simulink model "Ford_T3T6_ArchCnctnDigrm"  (R2016b)
settings: Solver=FixedStepDiscrete  StartTime=0.0  StopTime=10.0  RelTol=1e-3  EnableMultiTasking=on
libraries: canmsglib x15
(part 11 of 15)

== system Ford_T3T6_ArchCnctnDigrm/Vehicle Com/Rx Messages/Ambient Temperature ==
  note: FordVehOutdAirTVld Signal Required
  note: From COM
  MM078A_FordMsg41ABusHiSpd : Subsystem  Tag=4.0.X  Description=The purpose of the Ford Message 41A Bus High Speed function is to provide the Electric Power Steering system with vehicle odometer, climate, and Trailer Back Up Assist signals from CAN. The Ford Message 41A function will perform the missing message and signal invalid diagnostics as well as provide a validity signal for the signal values and received message.
      settings: AttributesFormatString=Version: %<Tag>
  Outside_Air_Temp_Stat : Ground
  tag scope: ComIPduCallout_Climate_Control_Data_FD1=global, ComTimeoutNotification_Outside_Air_Temp_Stat=global, FordVehOutdAirT=global, FordVehOutdAirTRaw=global
  wires:
  [ClrDiagcFlgProxy] -> MM078A_FordMsg41ABusHiSpd/1(ClrDiagcFlgProxy)
  [FordCanDtcInhb] -> MM078A_FordMsg41ABusHiSpd/2(FordCanDtcInhb)
  [FordEpsLifeCycMod] -> MM078A_FordMsg41ABusHiSpd/3(FordEpsLifeCycMod)
  Outside_Air_Temp_Stat/1 -> MM078A_FordMsg41ABusHiSpd/4(Ford_Outside_Air_Temp_Stat)
  [GetRefTmr100MicroSec32bit] -> MM078A_FordMsg41ABusHiSpd/5(GetRefTmr100MicroSec32bit)
  [GetTiSpan100MicroSec32bit] -> MM078A_FordMsg41ABusHiSpd/6(GetTiSpan100MicroSec32bit)
  [SetNtcSts] -> MM078A_FordMsg41ABusHiSpd/7(SetNtcSts)
  MM078A_FordMsg41ABusHiSpd/1(FordVehOutdAirT) -> [FordVehOutdAirT]
  MM078A_FordMsg41ABusHiSpd/2(FordVehOutdAirTRaw) -> [FordVehOutdAirTRaw]
  MM078A_FordMsg41ABusHiSpd/3(ComIPduCallout_Climate_Control_Data_FD1) -> [ComIPduCallout_Climate_Control_Data_FD1]
  MM078A_FordMsg41ABusHiSpd/4(ComTimeoutNotification_Outside_Air_Temp_Stat) -> [ComTimeoutNotification_Outside_Air_Temp_Stat]

== system Ford_T3T6_ArchCnctnDigrm/Vehicle Com/Rx Messages/Brake Data ==
  note: From COM
  note: From COM
  note: From COM
  note: From COM
  BrkTot_Tq_Actl : Ground
  Ground : Ground
  Ground6 : Ground
  Ground7 : Ground
  MM052A_FordMsg07DBusHiSpd : Subsystem  Tag=4.0.X  Description=The purpose of the Ford Message 07D Bus High Speed function is to provide the Electric Power Steering system with signal values for the Brake Oscillation Reduction and Trailer Back Up Assist function from CAN. The Ford Message 07D function will perform the missing message diagnostic, signal invalid diagnostic, and provide a validity flag for the received message and signal values.
      settings: AttributesFormatString=Version: %<Tag>
  MM058A_FordMsg165BusHiSpd : Subsystem  Tag=4.0.X  Description=The purpose of the Ford Message 165 Bus High Speed function is to provide the Electric Power Steering system with signal values for the EAC feature. The Ford Message 165 function will perform the missing message and signal invalid diagnostics.
      settings: AttributesFormatString=Version: %<Tag>
  MM063A_FordMsg213BusHiSpd : Subsystem  Tag=4.0.X  Description=The purpose of the Ford Message 213 Bus High Speed function is toprovide the Electric Power Steering system with signal values forthe Brake Oscillation Reduction, Lane Detection Warning, LKA, Traffic Jam Assist and Lane Center Assist functions from CAN.The FordMessage 213 function will perform the missing message and signal ivalid diagnostics as well as provide a validity flag for the signal values and received message.
      settings: AttributesFormatString=Version: %<Tag>
  MM077A_FordMsg415BusHiSpd : Subsystem  Tag=4.0.X  Description=The purpose of the Ford Message 415 Bus High Speed function is to provide the Electric Power Steering systemwith signal values for vehicle speed and the Trailer Back Up Assist function from CAN. The Ford Message 415function will perform the missing message and signal invalid diagnostics as well as provide a validity signalfor the signal values and received message.
      settings: AttributesFormatString=Version: %<Tag>
  VehVertComp_A_Actl : Ground
  tag scope: ComIPduCallout_BrakeSnData_4_FD1=global, ComIPduCallout_BrakeSysFeatures_FD1=global, ComIPduCallout_DesiredTorqBrk_FD1=global, ComIPduCallout_EngBrakeData_FD1=global, ComTimeoutNotification_BpedDrvAppl_D_Actl=global, ComTimeoutNotification_BrkTot_Tq_Actl=global, ComTimeoutNotification_CmbbDeny_B_ActlBrk=global, ComTimeoutNotification_Veh_V_ActlBrk=global, FordVehAbsActv=global, FordVehAbsEscStsVld=global, FordVehActBrkTqRaw=global, FordVehBrkPedlAppld=global, FordVehBrkPedlAppldQlyFac=global, FordVehBrkPedlVld=global, FordVehBrkTqVld=global, FordVehCllsnMtgtnByBrkgDenied=global, FordVehCllsnMtgtnByBrkgDisad=global, FordVehEscActv=global, FordVehLoSpdMtnCtrlBrkSprtSts=global, FordVehLoSpdMtnCtrlBrkSprtStsRaw=global, FordVehLoSpdMtnCtrlBrkSprtVld=global, FordVehSpdBrkModl=global, FordVehSpdBrkModlLoQlyVld=global, FordVehSpdBrkModlRaw=global, FordVehSpdBrkModlVld=global, FordVehSpdChksBrkModl=global, FordVehSpdCntrBrkModl=global, FordVehSpdQlyFacBrkModl=global, FordVehVertACmpdRaw=global, FordVehVertAVld=global
  wires:
  [ClrDiagcFlgProxy] -> MM052A_FordMsg07DBusHiSpd/1(ClrDiagcFlgProxy)
  [FordBrkOscnRednEnad] -> MM052A_FordMsg07DBusHiSpd/2(FordBrkOscnRednEnad)
  [FordCanDtcInhb] -> MM052A_FordMsg07DBusHiSpd/3(FordCanDtcInhb)
  [FordEpsLifeCycMod] -> MM052A_FordMsg07DBusHiSpd/4(FordEpsLifeCycMod)
  [FordTrlrBackupAssiEnad] -> MM052A_FordMsg07DBusHiSpd/5(FordTrlrBackUpAssiEnad)
  BrkTot_Tq_Actl/1 -> MM052A_FordMsg07DBusHiSpd/6(Ford_BrkTot_Tq_Actl)
  VehVertComp_A_Actl/1 -> MM052A_FordMsg07DBusHiSpd/7(Ford_VehVertComp_A_Actl)
  [GetRefTmr100MicroSec32bit] -> MM052A_FordMsg07DBusHiSpd/8(GetRefTmr100MicroSec32bit)
  [GetTiSpan100MicroSec32bit] -> MM052A_FordMsg07DBusHiSpd/9(GetTiSpan100MicroSec32bit)
  [SetNtcSts] -> MM052A_FordMsg07DBusHiSpd/10(SetNtcSts)
  MM052A_FordMsg07DBusHiSpd/1(FordVehActBrkTqRaw) -> [FordVehActBrkTqRaw]
  MM052A_FordMsg07DBusHiSpd/2(FordVehBrkTqVld) -> [FordVehBrkTqVld]
  MM052A_FordMsg07DBusHiSpd/3(FordVehVertACmpdRaw) -> [FordVehVertACmpdRaw]
  MM052A_FordMsg07DBusHiSpd/4(FordVehVertAVld) -> [FordVehVertAVld]
  MM052A_FordMsg07DBusHiSpd/5(ComIPduCallout_BrakeSnData_4_FD1) -> [ComIPduCallout_BrakeSnData_4_FD1]
  MM052A_FordMsg07DBusHiSpd/6(ComTimeoutNotification_BrkTot_Tq_Actl) -> [ComTimeoutNotification_BrkTot_Tq_Actl]
  [ClrDiagcFlgProxy] -> MM063A_FordMsg213BusHiSpd/1(ClrDiagcFlgProxy)
  [FordBrkOscnRednEnad] -> MM063A_FordMsg213BusHiSpd/2(FordBrkOscnRednEnad)
  [FordCanDtcInhb] -> MM063A_FordMsg213BusHiSpd/3(FordCanDtcInhb)
  [FordEpsLifeCycMod] -> MM063A_FordMsg213BusHiSpd/4(FordEpsLifeCycMod)
  [FordEvasSteerAssiEnad] -> MM063A_FordMsg213BusHiSpd/5(FordEvasSteerAssiEnad)
  [FordLaneCentrAssiEnad] -> MM063A_FordMsg213BusHiSpd/6(FordLaneCentrAssiEnad)
  [LaneDetnWarnEnad] -> MM063A_FordMsg213BusHiSpd/7(FordLaneDetnWarnEnad)
  [FordLaneKeepAssiEnad] -> MM063A_FordMsg213BusHiSpd/8(FordLkaEnad)
  [FordTrfcJamAssiEnad] -> MM063A_FordMsg213BusHiSpd/9(FordTrfcJamAssiEnad)
  Ground/1 -> MM063A_FordMsg213BusHiSpd/10(Ford_AbsActv_B_Actl1), MM063A_FordMsg213BusHiSpd/11(Ford_CmbbBrkDis_B_Actl1), MM063A_FordMsg213BusHiSpd/13(Ford_StabCtlBrkActv_B_Actl1), MM063A_FordMsg213BusHiSpd/12(Ford_CmbbDeny_B_ActlBrk1)
  [GetRefTmr100MicroSec32bit] -> MM063A_FordMsg213BusHiSpd/14(GetRefTmr100MicroSec32bit)
  [GetTiSpan100MicroSec32bit] -> MM063A_FordMsg213BusHiSpd/15(GetTiSpan100MicroSec32bit)
  [SetNtcSts] -> MM063A_FordMsg213BusHiSpd/16(SetNtcSts)
  MM063A_FordMsg213BusHiSpd/1(FordVehAbsActv) -> [FordVehAbsActv]
  MM063A_FordMsg213BusHiSpd/2(FordVehAbsEscStsVld) -> [FordVehAbsEscStsVld]
  MM063A_FordMsg213BusHiSpd/3(FordVehCllsnMtgtnByBrkgDenied) -> [FordVehCllsnMtgtnByBrkgDenied]
  MM063A_FordMsg213BusHiSpd/4(FordVehCllsnMtgtnByBrkgDisad) -> [FordVehCllsnMtgtnByBrkgDisad]
  MM063A_FordMsg213BusHiSpd/5(FordVehEscActv) -> [FordVehEscActv]
  MM063A_FordMsg213BusHiSpd/6(ComIPduCallout_DesiredTorqBrk_FD1) -> [ComIPduCallout_DesiredTorqBrk_FD1]
  MM063A_FordMsg213BusHiSpd/7(ComTimeoutNotification_CmbbDeny_B_ActlBrk) -> [ComTimeoutNotification_CmbbDeny_B_ActlBrk]
  [ClrDiagcFlgProxy] -> MM077A_FordMsg415BusHiSpd/1(ClrDiagcFlgProxy)
  [FordAbsPrsnt] -> MM077A_FordMsg415BusHiSpd/2(FordAbsPrsnt)
  [FordCanDtcInhb] -> MM077A_FordMsg415BusHiSpd/3(FordCanDtcInhb)
  [FordEpsLifeCycMod] -> MM077A_FordMsg415BusHiSpd/4(FordEpsLifeCycMod)
  [FordTrlrBackupAssiEnad] -> MM077A_FordMsg415BusHiSpd/5(FordTrlrBackupAssiEnad)
  Ground6/1 -> MM077A_FordMsg415BusHiSpd/6(Ford_LsmcBrkDecel_D_Stat1), MM077A_FordMsg415BusHiSpd/7(Ford_VehVActlBrk_D_Qf1), MM077A_FordMsg415BusHiSpd/8(Ford_VehVActlBrk_No_Cnt), MM077A_FordMsg415BusHiSpd/9(Ford_VehVActlBrk_No_Cs), MM077A_FordMsg415BusHiSpd/10(Ford_Veh_V_ActlBrk)
  [GetRefTmr100MicroSec32bit] -> MM077A_FordMsg415BusHiSpd/11(GetRefTmr100MicroSec32bit)
  [GetTiSpan100MicroSec32bit] -> MM077A_FordMsg415BusHiSpd/12(GetTiSpan100MicroSec32bit)
  [SetNtcSts] -> MM077A_FordMsg415BusHiSpd/13(SetNtcSts)
  MM077A_FordMsg415BusHiSpd/1(FordVehLoSpdMtnCtrlBrkSprtSts) -> [FordVehLoSpdMtnCtrlBrkSprtSts]
  MM077A_FordMsg415BusHiSpd/2(FordVehLoSpdMtnCtrlBrkSprtStsRaw) -> [FordVehLoSpdMtnCtrlBrkSprtStsRaw]
  MM077A_FordMsg415BusHiSpd/3(FordVehLoSpdMtnCtrlBrkSprtVld) -> [FordVehLoSpdMtnCtrlBrkSprtVld]
  MM077A_FordMsg415BusHiSpd/4(FordVehSpdBrkModl) -> [FordVehSpdBrkModl]
  MM077A_FordMsg415BusHiSpd/5(FordVehSpdBrkModlLoQlyVld) -> [FordVehSpdBrkModlLoQlyVld]
  MM077A_FordMsg415BusHiSpd/6(FordVehSpdBrkModlRaw) -> [FordVehSpdBrkModlRaw]
  MM077A_FordMsg415BusHiSpd/7(FordVehSpdBrkModlVld) -> [FordVehSpdBrkModlVld]
  MM077A_FordMsg415BusHiSpd/8(FordVehSpdChksBrkModl) -> [FordVehSpdChksBrkModl]
  MM077A_FordMsg415BusHiSpd/9(FordVehSpdCntrBrkModl) -> [FordVehSpdCntrBrkModl]
  MM077A_FordMsg415BusHiSpd/10(FordVehSpdQlyFacBrkModl) -> [FordVehSpdQlyFacBrkModl]
  MM077A_FordMsg415BusHiSpd/11(ComIPduCallout_BrakeSysFeatures_FD1) -> [ComIPduCallout_BrakeSysFeatures_FD1]
  MM077A_FordMsg415BusHiSpd/12(ComTimeoutNotification_Veh_V_ActlBrk) -> [ComTimeoutNotification_Veh_V_ActlBrk]
  [ClrDiagcFlgProxy] -> MM058A_FordMsg165BusHiSpd/1(ClrDiagcFlgProxy)
  [FordCanDtcInhb] -> MM058A_FordMsg165BusHiSpd/2(FordCanDtcInhb)
  [FordEpsLifeCycMod] -> MM058A_FordMsg165BusHiSpd/3(FordEpsLifeCycMod)
  [FordTrlrBackupAssiEnad] -> MM058A_FordMsg165BusHiSpd/4(FordTrlrBackupAssiEnad)
  Ground7/1 -> MM058A_FordMsg165BusHiSpd/5(Ford_BpedDrvAppl_D_Actl1), MM058A_FordMsg165BusHiSpd/6(Ford_BpedDrvAppl_D_Qf1)
  [GetRefTmr100MicroSec32bit] -> MM058A_FordMsg165BusHiSpd/7(GetRefTmr100MicroSec32bit)
  [GetTiSpan100MicroSec32bit] -> MM058A_FordMsg165BusHiSpd/8(GetTiSpan100MicroSec32bit)
  [SetNtcSts] -> MM058A_FordMsg165BusHiSpd/9(SetNtcSts)
  MM058A_FordMsg165BusHiSpd/1(FordVehBrkPedlAppld) -> [FordVehBrkPedlAppld]
  MM058A_FordMsg165BusHiSpd/2(FordVehBrkPedlAppldQlyFac) -> [FordVehBrkPedlAppldQlyFac]
  MM058A_FordMsg165BusHiSpd/3(FordVehBrkPedlVld) -> [FordVehBrkPedlVld]
  MM058A_FordMsg165BusHiSpd/4(ComIPduCallout_EngBrakeData_FD1) -> [ComIPduCallout_EngBrakeData_FD1]
  MM058A_FordMsg165BusHiSpd/5(ComTimeoutNotification_BpedDrvAppl_D_Actl) -> [ComTimeoutNotification_BpedDrvAppl_D_Actl]

== system Ford_T3T6_ArchCnctnDigrm/Vehicle Com/Rx Messages/Evasive Steer Assist ==
  note: Wrong in Component Requirements
  note: From COM
  note: From COM
  EsaOn_B_Rq : Ground
  Ground : Ground
  MM075A_FordMsg3D7BusHiSpd : Subsystem  Tag=4.0.X  Description=The purpose of the Ford Message 3D7 Bus High Speed function is to provide the Electric Power Steering system with signal values for the Evasive Steer Assist functions from CAN. The Ford Message 3D7 function will perform the missing message and signal invalid diagnostics as well as provide a validity flag for the signal values and received message.Detailed requirements have implemented the FordDBC file for guidance.
      settings: AttributesFormatString=Version: %<Tag>
  MM134A_FordMsg2FDBusHiSpd : Subsystem  Tag=4.0.X
      settings: AttributesFormatString=Version: %<Tag>
  tag scope: ComIPduCallout_Mc_Send_Signals_2_FD1=global, ComIPduCallout_Steer_Assist_Data_FD1=global, ComTimeoutNotification_EsaEnbl_D2_Rq=global, ComTimeoutNotification_EsaOn_B_Rq=global, FordVehCllsnMtgtnByBrkgLatDstRaw=global, FordVehCllsnMtgtnByBrkgLgtDstRaw=global, FordVehCllsnMtgtnByBrkgObjDataConfLvlRaw=global, FordVehCllsnMtgtnByBrkgObjTypClassnRaw=global, FordVehCllsnMtgtnByBrkgRelLatVelRaw=global, FordVehCllsnMtgtnByBrkgRelLgtVelRaw=global, FordVehCllsnMtgtnByBrkgTiToCllsnRaw=global, FordVehEvasSteerAssiEnadReqRaw=global, FordVehEvasSteerAssiImgProcrModlAVld=global, FordVehEvasSteerAssiReq=global, FordVehEvasSteerAssiReqVld=global
  wires:
  [ClrDiagcFlgProxy] -> MM134A_FordMsg2FDBusHiSpd/1(ClrDiagcFlgProxy)
  [FordCanDtcInhb] -> MM134A_FordMsg2FDBusHiSpd/2(FordCanDtcInhb)
  [FordEpsLifeCycMod] -> MM134A_FordMsg2FDBusHiSpd/3(FordEpsLifeCycMod)
  [FordInvldMsgDiagcInhb] -> MM134A_FordMsg2FDBusHiSpd/4(FordInvldMsgDiagcInhb)
  [FordMfgDiagcInhb] -> MM134A_FordMsg2FDBusHiSpd/5(FordMfgDiagcInhb)
  [FordMissMsgDiagcInhb] -> MM134A_FordMsg2FDBusHiSpd/6(FordMissMsgDiagcInhb)
  [FordTrlrBackupAssiEnad] -> MM134A_FordMsg2FDBusHiSpd/7(FordTrlrBackupAssiEnad)
  EsaOn_B_Rq/1 -> MM134A_FordMsg2FDBusHiSpd/8(Ford_EsaOn_B_Rq)
  [GetRefTmr100MicroSec32bit] -> MM134A_FordMsg2FDBusHiSpd/9(GetRefTmr100MicroSec32bit)
  [GetTiSpan100MicroSec32bit] -> MM134A_FordMsg2FDBusHiSpd/10(GetTiSpan100MicroSec32bit)
  [SetNtcSts] -> MM134A_FordMsg2FDBusHiSpd/11(SetNtcSts)
  MM134A_FordMsg2FDBusHiSpd/1(FordVehEvasSteerAssiReq) -> [FordVehEvasSteerAssiReq]
  MM134A_FordMsg2FDBusHiSpd/2(FordVehEvasSteerAssiReqVld) -> [FordVehEvasSteerAssiReqVld]
  MM134A_FordMsg2FDBusHiSpd/3(ComIPduCallout_Mc_Send_Signals_2_FD1) -> [ComIPduCallout_Mc_Send_Signals_2_FD1]
  MM134A_FordMsg2FDBusHiSpd/4(ComTimeoutNotification_EsaOn_B_Rq) -> [ComTimeoutNotification_EsaOn_B_Rq]
  [ClrDiagcFlgProxy] -> MM075A_FordMsg3D7BusHiSpd/1(ClrDiagcFlgProxy)
  [FordCanDtcInhb] -> MM075A_FordMsg3D7BusHiSpd/2(FordCanDtcInhb)
  [FordEpsLifeCycMod] -> MM075A_FordMsg3D7BusHiSpd/3(FordEpsLifeCycMod)
  [FordEvasSteerAssiEnad] -> MM075A_FordMsg3D7BusHiSpd/4(FordEvasSteerAssiEnad)
  Ground/1 -> MM075A_FordMsg3D7BusHiSpd/12(Ford_EsaEnbl_D2_Rq1), MM075A_FordMsg3D7BusHiSpd/11(Ford_CmbbObjRelLong_V_Actl), MM075A_FordMsg3D7BusHiSpd/10(Ford_CmbbObjRelLat_V_Actl), MM075A_FordMsg3D7BusHiSpd/9(Ford_CmbbObjDistLong_L_Actl), MM075A_FordMsg3D7BusHiSpd/8(Ford_CmbbObjDistLat_L_Actl), MM075A_FordMsg3D7BusHiSpd/7(Ford_CmbbObjConfdnc_D_Stat1), MM075A_FordMsg3D7BusHiSpd/6(Ford_CmbbObjColl_T_Actl), MM075A_FordMsg3D7BusHiSpd/5(Ford_CmbbObjClass_D_Stat1)
  [GetRefTmr100MicroSec32bit] -> MM075A_FordMsg3D7BusHiSpd/13(GetRefTmr100MicroSec32bit)
  [GetTiSpan100MicroSec32bit] -> MM075A_FordMsg3D7BusHiSpd/14(GetTiSpan100MicroSec32bit)
  [SetNtcSts] -> MM075A_FordMsg3D7BusHiSpd/15(SetNtcSts)
  MM075A_FordMsg3D7BusHiSpd/1(FordVehCllsnMtgtnByBrkgLatDstRaw) -> [FordVehCllsnMtgtnByBrkgLatDstRaw]
  MM075A_FordMsg3D7BusHiSpd/2(FordVehCllsnMtgtnByBrkgLgtDstRaw) -> [FordVehCllsnMtgtnByBrkgLgtDstRaw]
  MM075A_FordMsg3D7BusHiSpd/3(FordVehCllsnMtgtnByBrkgObjDataConfLvlRaw) -> [FordVehCllsnMtgtnByBrkgObjDataConfLvlRaw]
  MM075A_FordMsg3D7BusHiSpd/4(FordVehCllsnMtgtnByBrkgObjTypClassnRaw) -> [FordVehCllsnMtgtnByBrkgObjTypClassnRaw]
  MM075A_FordMsg3D7BusHiSpd/5(FordVehCllsnMtgtnByBrkgRelLatVelRaw) -> [FordVehCllsnMtgtnByBrkgRelLatVelRaw]
  MM075A_FordMsg3D7BusHiSpd/6(FordVehCllsnMtgtnByBrkgRelLgtVelRaw) -> [FordVehCllsnMtgtnByBrkgRelLgtVelRaw]
  MM075A_FordMsg3D7BusHiSpd/7(FordVehCllsnMtgtnByBrkgTiToCllsnRaw) -> [FordVehCllsnMtgtnByBrkgTiToCllsnRaw]
  MM075A_FordMsg3D7BusHiSpd/8(FordVehEvasSteerAssiEnadReqRaw) -> [FordVehEvasSteerAssiEnadReqRaw]
  MM075A_FordMsg3D7BusHiSpd/9(FordVehEvasSteerAssiImgProcrModlAVld) -> [FordVehEvasSteerAssiImgProcrModlAVld]
  MM075A_FordMsg3D7BusHiSpd/10(ComIPduCallout_Steer_Assist_Data_FD1) -> [ComIPduCallout_Steer_Assist_Data_FD1]
  MM075A_FordMsg3D7BusHiSpd/11(ComTimeoutNotification_EsaEnbl_D2_Rq) -> [ComTimeoutNotification_EsaEnbl_D2_Rq]

== system Ford_T3T6_ArchCnctnDigrm/Vehicle Com/Rx Messages/Lane Keep Asssist ==
  note: From COM
  LaCurvature_No_Calc : Ground
  MM073A_FordMsg3CABusHiSpd : Subsystem  Tag=4.0.X  Description=The purpose of the Ford Message 3CA Bus Hish Speed function isto provide the Electric Power Steering system with signal values for Lane Detection Warning and Lane Keep Assist functions form CAN.The Ford Message 3CA function will perform the missing message and signal invalid diagnostics as well as provide a validity signal for the signal values and received message.
      settings: AttributesFormatString=Version: %<Tag>
  tag scope: ComIPduCallout_Lane_Assist_Data1_FD1=global, ComTimeoutNotification_LaCurvature_No_Calc=global, FordVehLaneAssiImgProcgModlAVld=global, FordVehLaneDetnWarnInten=global, FordVehLaneDetnWarnSts=global, FordVehLaneKeepSysCrvt=global, FordVehLaneKeepSysCrvtRaw=global, FordVehLaneKeepSysRampTyp=global, FordVehLaneKeepSysReqdAg=global, FordVehLaneKeepSysReqdAgRaw=global, FordVehLaneKeepSysSts=global
  wires:
  [ClrDiagcFlgProxy] -> MM073A_FordMsg3CABusHiSpd/1(ClrDiagcFlgProxy)
  [FordCanDtcInhb] -> MM073A_FordMsg3CABusHiSpd/2(FordCanDtcInhb)
  [FordEpsLifeCycMod] -> MM073A_FordMsg3CABusHiSpd/3(FordEpsLifeCycMod)
  [LaneDetnWarnEnad] -> MM073A_FordMsg3CABusHiSpd/4(FordLaneDetnWarnEnad)
  [FordLaneKeepAssiEnad] -> MM073A_FordMsg3CABusHiSpd/5(FordLaneKeepAssiEnad)
  LaCurvature_No_Calc/1 -> MM073A_FordMsg3CABusHiSpd/7(Ford_LaRampType_B_Req1), MM073A_FordMsg3CABusHiSpd/10(Ford_LdwActvStats_D_Req1), MM073A_FordMsg3CABusHiSpd/11(Ford_LkaActvStats_D2_Req1), MM073A_FordMsg3CABusHiSpd/9(Ford_LdwActvIntns_D_Req1), MM073A_FordMsg3CABusHiSpd/8(Ford_LaRefAng_No_Req), MM073A_FordMsg3CABusHiSpd/6(Ford_LaCurvature_No_Calc)
  [GetRefTmr100MicroSec32bit] -> MM073A_FordMsg3CABusHiSpd/12(GetRefTmr100MicroSec32bit)
  [GetTiSpan100MicroSec32bit] -> MM073A_FordMsg3CABusHiSpd/13(GetTiSpan100MicroSec32bit)
  [SetNtcSts] -> MM073A_FordMsg3CABusHiSpd/14(SetNtcSts)
  MM073A_FordMsg3CABusHiSpd/1(FordVehLaneAssiImgProcgModlAVld) -> [FordVehLaneAssiImgProcgModlAVld]
  MM073A_FordMsg3CABusHiSpd/2(FordVehLaneDetnWarnInten) -> [FordVehLaneDetnWarnInten]
  MM073A_FordMsg3CABusHiSpd/3(FordVehLaneDetnWarnSts) -> [FordVehLaneDetnWarnSts]
  MM073A_FordMsg3CABusHiSpd/4(FordVehLaneKeepSysCrvt) -> [FordVehLaneKeepSysCrvt]
  MM073A_FordMsg3CABusHiSpd/5(FordVehLaneKeepSysCrvtRaw) -> [FordVehLaneKeepSysCrvtRaw]
  MM073A_FordMsg3CABusHiSpd/6(FordVehLaneKeepSysRampTyp) -> [FordVehLaneKeepSysRampTyp]
  MM073A_FordMsg3CABusHiSpd/7(FordVehLaneKeepSysReqdAg) -> [FordVehLaneKeepSysReqdAg]
  MM073A_FordMsg3CABusHiSpd/8(FordVehLaneKeepSysReqdAgRaw) -> [FordVehLaneKeepSysReqdAgRaw]
  MM073A_FordMsg3CABusHiSpd/9(FordVehLaneKeepSysSts) -> [FordVehLaneKeepSysSts]
  MM073A_FordMsg3CABusHiSpd/10(ComIPduCallout_Lane_Assist_Data1_FD1) -> [ComIPduCallout_Lane_Assist_Data1_FD1]
  MM073A_FordMsg3CABusHiSpd/11(ComTimeoutNotification_LaCurvature_No_Calc) -> [ComTimeoutNotification_LaCurvature_No_Calc]

== system Ford_T3T6_ArchCnctnDigrm/Vehicle Com/Rx Messages/Lat and Long Acceleration ==
  note: From COM
  note: From COM
  Ground14 : Ground
  "HandsOffCnfm_B_Rq " : Ground
  LatCtlCurv_NoRate_Actl : Ground
  LatCtlCurv_No_Actl : Ground
  LatCtlPathOffst_L_Actl : Ground
  LatCtlPath_An_Actl : Ground
  LatCtlPrecision_D_Rq : Ground
  LatCtlRampType_D_Rq : Ground
  LatCtlRng_L_Max : Ground
  LatCtl_D_Rq : Ground
  MM074A_FordMsg3D3BusHiSpd : Subsystem  Tag=1.0.0  Description=The purpose of the Ford Message 3D3 Bus High Speed function is to provide the Electric Power Steering system with signal values for the Traffic Jam Assist and Lane Center Assist functions from CAN. The Ford Message 3D3 function will perform the missing message as well as provide a validity flag for the signal values and received message.
      settings: AttributesFormatString=Version: %<Tag>
  MM124A_FordMsg077BusHiSpd1 : Subsystem  Tag=1.0.X  Description=The purpose of the Ford Message 077 Bus High Speed function is to provide the Electric Power Steering system with signal values for the Torque Steer Compensation, Brake Oscillation Reduction, Lane Keep Assist, Traffic Jam Assist, Lane Centering Assist, Pull Drift Compensation, Trailer Backup Assistance, and Evasive Steering Assist function from CAN. The Ford Message 077 function will perform the missing message and signal invalid diagnostics as well as provide a validity flag for the signal values and received message.
      settings: AttributesFormatString=Version: %<Tag>
  tag scope: ComIPduCallout_BrakeSnData_3_FD1=global, ComTimeoutNotification_VehLatComp_A_Actl=global, FordMsg3D3HiSpdBusClrDiagcSrv=global, FordMsg3D3HiSpdBusSerlComInpDi=global, FordVehLatACmpd=global, FordVehLatACmpdRaw=global, FordVehLatACmpdVld=global, FordVehLatCtrlCrvt=global, FordVehLatCtrlCrvtRate=global, FordVehLatCtrlCrvtRateRaw=global, FordVehLatCtrlCrvtRaw=global, FordVehLatCtrlHandsOffDetnTqStimlsReq=global, FordVehLatCtrlImgProcrModlAVld=global, FordVehLatCtrlPah=global, FordVehLatCtrlPahOffs=global, FordVehLatCtrlPahOffsRaw=global, FordVehLatCtrlPahRaw=global, FordVehLatCtrlPrcsn=global, FordVehLatCtrlRampTyp=global, FordVehLatCtrlReq=global, FordVehLatCtrlRingMax=global, FordVehLgtACmpd=global, FordVehLgtACmpdRaw=global, FordVehLgtACmpdVld=global, FordVehSpdOverGnd=global, FordVehSpdOverGndRaw=global, FordVehSpdOverGndVld=global, FordVehYawRateCmpd=global, FordVehYawRateCmpdRaw=global, FordVehYawRateCmpdVld=global
  wires:
  [FordCanDtcInhb] -> MM074A_FordMsg3D3BusHiSpd/1(CanDtcInhb)
  [FordEpsLifeCycMod] -> MM074A_FordMsg3D3BusHiSpd/2(EpsLifeCycMod)
  [FordLaneCentrAssiEnad] -> MM074A_FordMsg3D3BusHiSpd/3(LaneCentrAssiEnad)
  LatCtlCurv_No_Actl/1 -> MM074A_FordMsg3D3BusHiSpd/4(LatCtrlCrvt)
  LatCtlCurv_NoRate_Actl/1 -> MM074A_FordMsg3D3BusHiSpd/5(LatCtrlCrvtRate)
  "HandsOffCnfm_B_Rq "/1 -> MM074A_FordMsg3D3BusHiSpd/6(LatCtrlHandsOffDetnTqStimlsReq)
  LatCtlPath_An_Actl/1 -> MM074A_FordMsg3D3BusHiSpd/7(LatCtrlPah)
  LatCtlPathOffst_L_Actl/1 -> MM074A_FordMsg3D3BusHiSpd/8(LatCtrlPahOffs)
  LatCtlPrecision_D_Rq/1 -> MM074A_FordMsg3D3BusHiSpd/9(LatCtrlPrcsn)
  LatCtlRampType_D_Rq/1 -> MM074A_FordMsg3D3BusHiSpd/10(LatCtrlRampTyp)
  LatCtl_D_Rq/1 -> MM074A_FordMsg3D3BusHiSpd/11(LatCtrlReq)
  LatCtlRng_L_Max/1 -> MM074A_FordMsg3D3BusHiSpd/12(LatCtrlRingMax)
  [FordMissMsgDiagcInhb] -> MM074A_FordMsg3D3BusHiSpd/13(MissMsg3D3TiFlg)
  [FordTrfcJamAssiEnad] -> MM074A_FordMsg3D3BusHiSpd/14(TrfcJamAssiEnad)
  [GetRefTmr100MicroSec32bit] -> MM074A_FordMsg3D3BusHiSpd/15(GetRefTmr100MicroSec32bit)
  [GetTiSpan100MicroSec32bit] -> MM074A_FordMsg3D3BusHiSpd/16(GetTiSpan100MicroSec32bit)
  [SetNtcSts] -> MM074A_FordMsg3D3BusHiSpd/17(SetNtcSts)
  MM074A_FordMsg3D3BusHiSpd/1(FordVehLatCtrlCrvt) -> [FordVehLatCtrlCrvt]
  MM074A_FordMsg3D3BusHiSpd/2(FordVehLatCtrlCrvtRate) -> [FordVehLatCtrlCrvtRate]
  MM074A_FordMsg3D3BusHiSpd/3(FordVehLatCtrlCrvtRateRaw) -> [FordVehLatCtrlCrvtRateRaw]
  MM074A_FordMsg3D3BusHiSpd/4(FordVehLatCtrlCrvtRaw) -> [FordVehLatCtrlCrvtRaw]
  MM074A_FordMsg3D3BusHiSpd/5(FordVehLatCtrlHandsOffDetnTqStimlsReq) -> [FordVehLatCtrlHandsOffDetnTqStimlsReq]
  MM074A_FordMsg3D3BusHiSpd/6(FordVehLatCtrlImgProcrModlAVld) -> [FordVehLatCtrlImgProcrModlAVld]
  MM074A_FordMsg3D3BusHiSpd/7(FordVehLatCtrlPah) -> [FordVehLatCtrlPah]
  MM074A_FordMsg3D3BusHiSpd/8(FordVehLatCtrlPahOffs) -> [FordVehLatCtrlPahOffs]
  MM074A_FordMsg3D3BusHiSpd/9(FordVehLatCtrlPahOffsRaw) -> [FordVehLatCtrlPahOffsRaw]
  MM074A_FordMsg3D3BusHiSpd/10(FordVehLatCtrlPahRaw) -> [FordVehLatCtrlPahRaw]
  MM074A_FordMsg3D3BusHiSpd/11(FordVehLatCtrlPrcsn) -> [FordVehLatCtrlPrcsn]
  MM074A_FordMsg3D3BusHiSpd/12(FordVehLatCtrlRampTyp) -> [FordVehLatCtrlRampTyp]
  MM074A_FordMsg3D3BusHiSpd/13(FordVehLatCtrlReq) -> [FordVehLatCtrlReq]
  MM074A_FordMsg3D3BusHiSpd/14(FordVehLatCtrlRingMax) -> [FordVehLatCtrlRingMax]
  MM074A_FordMsg3D3BusHiSpd/15(FordMsg3D3HiSpdBusClrDiagcSrv) -> [FordMsg3D3HiSpdBusClrDiagcSrv]
  MM074A_FordMsg3D3BusHiSpd/16(FordMsg3D3HiSpdBusSerlComInpDi) -> [FordMsg3D3HiSpdBusSerlComInpDi]
  [FordBrkOscnRednEnad] -> MM124A_FordMsg077BusHiSpd1/1(FordBrkOscnRednEnad)
  [FordCanDtcInhb] -> MM124A_FordMsg077BusHiSpd1/2(FordCanDtcInhb)
  [FordEpsLifeCycMod] -> MM124A_FordMsg077BusHiSpd1/3(FordEpsLifeCycMod)
  [FordEvasSteerAssiEnad] -> MM124A_FordMsg077BusHiSpd1/4(FordEvasSteerAssiEnad)
  [FordLaneKeepAssiEnad] -> MM124A_FordMsg077BusHiSpd1/5(FordLaneKeepingAssiEnad)
  [FordMissMsgDiagcInhb] -> MM124A_FordMsg077BusHiSpd1/6(FordMissMsgDiagcInhb)
  [FordPullDriftCmpEnad] -> MM124A_FordMsg077BusHiSpd1/7(FordPullDriftCmpEnad)
  [FordTqSteerCmpEnad] -> MM124A_FordMsg077BusHiSpd1/8(FordTqSteerCmpEnad)
  [FordTrlrBackupAssiEnad] -> MM124A_FordMsg077BusHiSpd1/9(FordTrlrBackupAssiEnad)
  Ground14/1 -> MM124A_FordMsg077BusHiSpd1/12(Ford_VehOverGnd_V_Est), MM124A_FordMsg077BusHiSpd1/13(Ford_VehYawComp_W_Actl), MM124A_FordMsg077BusHiSpd1/11(Ford_VehLongComp_A_Actl), MM124A_FordMsg077BusHiSpd1/10(Ford_VehLatComp_A_Actl)
  [FordLaneCentrAssiEnad] -> MM124A_FordMsg077BusHiSpd1/14(LaneCentrAssiEnad)
  [FordTrfcJamAssiEnad] -> MM124A_FordMsg077BusHiSpd1/15(TrfcJamAssiEnad)
  [GetRefTmr100MicroSec32bit] -> MM124A_FordMsg077BusHiSpd1/16(GetRefTmr100MicroSec32bit)
  [GetTiSpan100MicroSec32bit] -> MM124A_FordMsg077BusHiSpd1/17(GetTiSpan100MicroSec32bit)
  [SetNtcSts] -> MM124A_FordMsg077BusHiSpd1/18(SetNtcSts)
  MM124A_FordMsg077BusHiSpd1/1(FordVehLatACmpd) -> [FordVehLatACmpd]
  MM124A_FordMsg077BusHiSpd1/2(FordVehLatACmpdRaw) -> [FordVehLatACmpdRaw]
  MM124A_FordMsg077BusHiSpd1/3(FordVehLatACmpdVld) -> [FordVehLatACmpdVld]
  MM124A_FordMsg077BusHiSpd1/4(FordVehLgtACmpd) -> [FordVehLgtACmpd]
  MM124A_FordMsg077BusHiSpd1/5(FordVehLgtACmpdRaw) -> [FordVehLgtACmpdRaw]
  MM124A_FordMsg077BusHiSpd1/6(FordVehLgtACmpdVld) -> [FordVehLgtACmpdVld]
  MM124A_FordMsg077BusHiSpd1/7(FordVehSpdOverGnd) -> [FordVehSpdOverGnd]
  MM124A_FordMsg077BusHiSpd1/8(FordVehSpdOverGndRaw) -> [FordVehSpdOverGndRaw]
  MM124A_FordMsg077BusHiSpd1/9(FordVehSpdOverGndVld) -> [FordVehSpdOverGndVld]
  MM124A_FordMsg077BusHiSpd1/10(FordVehYawRateCmpd) -> [FordVehYawRateCmpd]
  MM124A_FordMsg077BusHiSpd1/11(FordVehYawRateCmpdRaw) -> [FordVehYawRateCmpdRaw]
  MM124A_FordMsg077BusHiSpd1/12(FordVehYawRateCmpdVld) -> [FordVehYawRateCmpdVld]
  MM124A_FordMsg077BusHiSpd1/13(ComIPduCallout_BrakeSnData_3_FD1) -> [ComIPduCallout_BrakeSnData_3_FD1]
  MM124A_FordMsg077BusHiSpd1/14(ComTimeoutNotification_VehLatComp_A_Actl) -> [ComTimeoutNotification_VehLatComp_A_Actl]

== system Ford_T3T6_ArchCnctnDigrm/Vehicle Com/Rx Messages/Park Assist ==
  note: From COM
  Ground : Ground
  Ground1 : Ground
  Ground2 : Ground
  MM071A_FordMsg3A8BusHiSpd : Subsystem  Tag=4.0.X  Description=The purpose of the Ford Message 3A8 Bus High Speed function is to providethe Electric Power Steering system with signal values for the APA,External Angle Control and Trailer Back Up Assist functions from CAN.The Ford Message 3A8 function will perform the missing message and signalinvalid diagnostics as well as provide a validity flag for the signal values and received message.
      settings: AttributesFormatString=Version: %<Tag>
  tag scope: ComIPduCallout_ParkAid_Data_FD1=global, ComTimeoutNotification_EPASExtAngleStatReq=global, FordVehParkAidModlReqdAg=global, FordVehParkAidModlReqdAgRaw=global, FordVehParkAidModlReqdAgVldInt=global, FordVehParkAidModlReqdSts=global, FordVehParkAidModlStsVld=global, FordVehParkAidModlStsVldInt=global, FordVehParkAidModlSysSt=global
  wires:
  [ClrDiagcFlgProxy] -> MM071A_FordMsg3A8BusHiSpd/1(ClrDiagcFlgProxy)
  [FordActvParkAssiEnad] -> MM071A_FordMsg3A8BusHiSpd/2(FordApaEnad)
  [FordCanDtcInhb] -> MM071A_FordMsg3A8BusHiSpd/3(FordCanDtcInhb)
  [FordEpsLifeCycMod] -> MM071A_FordMsg3A8BusHiSpd/4(FordEpsLifeCycMod)
  [FordExtAgCtrlEnad] -> MM071A_FordMsg3A8BusHiSpd/5(FordExtAgCtrlEnad)
  [FordTrlrBackupAssiEnad] -> MM071A_FordMsg3A8BusHiSpd/6(FordTrlrBackUpAssiEnad)
  Ground/1 -> MM071A_FordMsg3A8BusHiSpd/7(Ford_ApaSys_D_Stat1)
  Ground1/1 -> MM071A_FordMsg3A8BusHiSpd/8(Ford_EPASExtAngleStatReq1)
  Ground2/1 -> MM071A_FordMsg3A8BusHiSpd/9(Ford_ExtSteeringAngleReq2)
  [GetRefTmr100MicroSec32bit] -> MM071A_FordMsg3A8BusHiSpd/10(GetRefTmr100MicroSec32bit)
  [GetTiSpan100MicroSec32bit] -> MM071A_FordMsg3A8BusHiSpd/11(GetTiSpan100MicroSec32bit)
  [SetNtcSts] -> MM071A_FordMsg3A8BusHiSpd/12(SetNtcSts)
  MM071A_FordMsg3A8BusHiSpd/1(FordVehParkAidModlReqdAg) -> [FordVehParkAidModlReqdAg]
  MM071A_FordMsg3A8BusHiSpd/2(FordVehParkAidModlReqdAgRaw) -> [FordVehParkAidModlReqdAgRaw]
  MM071A_FordMsg3A8BusHiSpd/3(FordVehParkAidModlReqdAgVldInt) -> [FordVehParkAidModlReqdAgVldInt]
  MM071A_FordMsg3A8BusHiSpd/4(FordVehParkAidModlReqdSts) -> [FordVehParkAidModlReqdSts]
  MM071A_FordMsg3A8BusHiSpd/5(FordVehParkAidModlStsVld) -> [FordVehParkAidModlStsVld]
  MM071A_FordMsg3A8BusHiSpd/6(FordVehParkAidModlStsVldInt) -> [FordVehParkAidModlStsVldInt]
  MM071A_FordMsg3A8BusHiSpd/7(FordVehParkAidModlSysSt) -> [FordVehParkAidModlSysSt]
  MM071A_FordMsg3A8BusHiSpd/8(ComIPduCallout_ParkAid_Data_FD1) -> [ComIPduCallout_ParkAid_Data_FD1]
  MM071A_FordMsg3A8BusHiSpd/9(ComTimeoutNotification_EPASExtAngleStatReq) -> [ComTimeoutNotification_EPASExtAngleStatReq]

== system Ford_T3T6_ArchCnctnDigrm/Vehicle Com/Rx Messages/Pinion Data ==
  note: From COM
  Ground3 : Ground
  MM070A_FordMsg414BusHiSpd : Subsystem  Tag=2.0.0  Description=The purpose of the Ford Message 414 Bus High Speed function isto provide the Electric Power Steering system with signal valuesfor base electric power steering functionalityDetailed requirements have implemented the Ford DBC file for guidance.
      settings: AttributesFormatString=Version: %<Tag>
  tag scope: ComIPduCallout_BrakeSnData_6_HS2=global, ComTimeoutNotification_Ford_StePinOffst_D_Stat=global, FordVehSteerPinionAgOffs=global, FordVehSteerPinionAgOffsRaw=global, FordVehSteerPinionAgOffsVld=global, FordVehSteerPinionOffsChks=global, FordVehSteerPinionOffsCnt=global, FordVehSteerPinionOffsSts=global, FordVehSteerPinionOffsStsRaw=global
  wires:
  Ground3/1 -> MM070A_FordMsg414BusHiSpd/4(Ford_StePinOffst_No_Cs), MM070A_FordMsg414BusHiSpd/3(Ford_StePinOffst_No_Cnt), MM070A_FordMsg414BusHiSpd/2(Ford_StePinOffst_D_Stat1), MM070A_FordMsg414BusHiSpd/1(Ford_StePinOffst_An_Est)
  [GetRefTmr100MicroSec32bit] -> MM070A_FordMsg414BusHiSpd/5(GetRefTmr100MicroSec32bit)
  [GetTiSpan100MicroSec32bit] -> MM070A_FordMsg414BusHiSpd/6(GetTiSpan100MicroSec32bit)
  MM070A_FordMsg414BusHiSpd/1(FordVehSteerPinionAgOffs) -> [FordVehSteerPinionAgOffs]
  MM070A_FordMsg414BusHiSpd/2(FordVehSteerPinionAgOffsRaw) -> [FordVehSteerPinionAgOffsRaw]
  MM070A_FordMsg414BusHiSpd/3(FordVehSteerPinionAgOffsVld) -> [FordVehSteerPinionAgOffsVld]
  MM070A_FordMsg414BusHiSpd/4(FordVehSteerPinionOffsChks) -> [FordVehSteerPinionOffsChks]
  MM070A_FordMsg414BusHiSpd/5(FordVehSteerPinionOffsCnt) -> [FordVehSteerPinionOffsCnt]
  MM070A_FordMsg414BusHiSpd/6(FordVehSteerPinionOffsSts) -> [FordVehSteerPinionOffsSts]
  MM070A_FordMsg414BusHiSpd/7(FordVehSteerPinionOffsStsRaw) -> [FordVehSteerPinionOffsStsRaw]
  MM070A_FordMsg414BusHiSpd/8(ComIPduCallout_BrakeSnData_6_HS2) -> [ComIPduCallout_BrakeSnData_6_HS2]
  MM070A_FordMsg414BusHiSpd/9(ComTimeoutNotification_Ford_StePinOffst_D_Stat) -> [ComTimeoutNotification_Ford_StePinOffst_D_Stat]

== system Ford_T3T6_ArchCnctnDigrm/Vehicle Com/Rx Messages/Steering Request Command ==
  note: From COM
  Ground3 : Ground
  MM123A_FordMsg076BusHiSpd1 : Subsystem  Tag=0.0.X
      settings: AttributesFormatString=Version: %<Tag>
  tag scope: ComIPduCallout_BrakeSnData_5_FD1=global, ComTimeoutNotification_DrvSte_Tq_Rq=global, FordVehDrvrSteerReqCmd=global, FordVehDrvrSteerReqCmdVld=global, FordVehDrvrSteerReqSts=global
  wires:
  [ClrDiagcFlgProxy] -> MM123A_FordMsg076BusHiSpd1/1(ClrDiagcFlgProxy)
  [DrvrSteerRcmdnEnad] -> MM123A_FordMsg076BusHiSpd1/2(DrvrSteerRcmdnEnad)
  [FordCanDtcInhb] -> MM123A_FordMsg076BusHiSpd1/3(FordCanDtcInhb)
  [FordEpsLifeCycMod] -> MM123A_FordMsg076BusHiSpd1/4(FordEpsLifeCycMod)
  Ground3/1 -> MM123A_FordMsg076BusHiSpd1/6(Ford_DrvSte_Tq_Rq), MM123A_FordMsg076BusHiSpd1/5(Ford_DrvSte_D_Stat)
  [GetRefTmr100MicroSec32bit] -> MM123A_FordMsg076BusHiSpd1/7(GetRefTmr100MicroSec32bit)
  [GetTiSpan100MicroSec32bit] -> MM123A_FordMsg076BusHiSpd1/8(GetTiSpan100MicroSec32bit)
  [SetNtcSts] -> MM123A_FordMsg076BusHiSpd1/9(SetNtcSts)
  MM123A_FordMsg076BusHiSpd1/1(FordVehDrvrSteerReqCmd) -> [FordVehDrvrSteerReqCmd]
  MM123A_FordMsg076BusHiSpd1/2(FordVehDrvrSteerReqCmdVld) -> [FordVehDrvrSteerReqCmdVld]
  MM123A_FordMsg076BusHiSpd1/3(FordVehDrvrSteerReqSts) -> [FordVehDrvrSteerReqSts]
  MM123A_FordMsg076BusHiSpd1/4(ComIPduCallout_BrakeSnData_5_FD1) -> [ComIPduCallout_BrakeSnData_5_FD1]
  MM123A_FordMsg076BusHiSpd1/5(ComTimeoutNotification_DrvSte_Tq_Rq) -> [ComTimeoutNotification_DrvSte_Tq_Rq]
